simulink model "open_loop_system_modal_kp_kv_int_robustness"  (R2018b)
settings: Solver=ode45  StartTime=0.0  StopTime=10  RelTol=1e-3  EnableMultiTasking=on
values from neighbouring files (symbols this model uses):
  Jpl = 0.0124    [lead_compensator.m]    (also in open_loop_complete_system_analysis.m; poles_placement_kp_kv.m; poles_placement_kp_kv_int.m)
  k = 1    [lead_compensator.m]    (also in poles_placement_kp_kv.m = place(openloop_modal_ss.a,openloop_modal_ss.b,lambda); poles_placement_kp_kv_int.m = place(openloop_modal_int_ss.a,openloop_modal_int_ss.b,lambda)
  km = 0.0235    [lead_compensator.m]    (also in open_loop_complete_system_analysis.m; poles_placement_kp_kv.m; poles_placement_kp_kv_int.m)
settings Model: Creator=c.ponzoni  LastModifiedBy=c.ponzoni
settings DataIOCC: LimitDataPoints=on  SaveFormat=Array
settings OptimizationCC: ExpressionDepthLimit=2147483647  LifeSpan=inf
settings DebuggingCC: UnderspecifiedInitializationDetection=Classic  MergeDetectMultiDrivingBlocksExec=none  StateNameClashWarn=warning  SFUnexpectedBacktrackingDiag=warning  SFNoUnconditionalDefaultTransitionDiag=warning  SFExecutionAtInitializationDiag=none
settings HardwareCC: ProdBitPerPointer=32  ProdBitPerSizeT=32  ProdBitPerPtrDiffT=32  ProdLargestAtomicFloat=None  ProdIntDivRoundTo=Undefined  ProdEndianess=Unspecified  ProdWordSize=32  ProdHWDeviceType=32-bit Generic
settings ModelReferenceCC: PropagateSignalLabelsOutOfModel=off
settings SFSimCC: SimUseLocalCustomCode=off
settings RTWCC: RTWUseLocalCustomCode=off
settings CodeAppCC: StateflowObjectComments=on
settings GRTTargetCC: TargetLangStandard=C89/C90 (ANSI)  GeneratePreprocessorConditionals=Disable all
settings ConfigComp: CovMetricSettings=dw  CovHtmlReporting=on  CovSaveCumulativeToWorkspaceVar=on  CovSaveSingleToWorkspaceVar=on  CovExternalEMLEnable=off

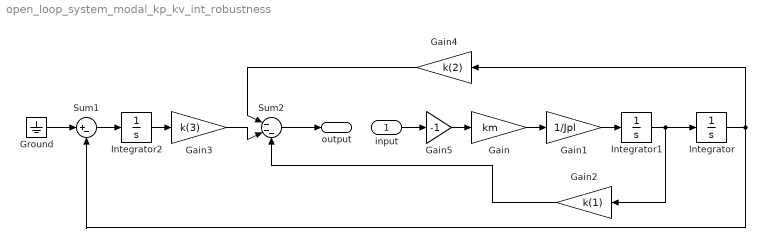
== system open_loop_system_modal_kp_kv_int_robustness ==
  input : Inport
  Gain : Gain  Gain=km  SaturateOnIntegerOverflow=on  OutDataTypeStr=Inherit: Same as input  ParamDataTypeStr=Inherit: Same as input
  Gain1 : Gain  Gain=1/Jpl  SaturateOnIntegerOverflow=on  OutDataTypeStr=Inherit: Same as input  ParamDataTypeStr=Inherit: Same as input
  Gain2 : Gain  Gain=k(1)  SaturateOnIntegerOverflow=on  OutDataTypeStr=Inherit: Same as input  ParamDataTypeStr=Inherit: Same as input
  Gain3 : Gain  Gain=k(3)  SaturateOnIntegerOverflow=on  OutDataTypeStr=Inherit: Same as input  ParamDataTypeStr=Inherit: Same as input
  Gain4 : Gain  Gain=k(2)  SaturateOnIntegerOverflow=on  OutDataTypeStr=Inherit: Same as input  ParamDataTypeStr=Inherit: Same as input
  Gain5 : Gain  Gain=-1  SaturateOnIntegerOverflow=on  OutDataTypeStr=Inherit: Same as input  ParamDataTypeStr=Inherit: Same as input
  Ground : Ground
  Integrator : Integrator
  Integrator1 : Integrator
  Integrator2 : Integrator
  Sum1 : Sum  Inputs=|+-
  Sum2 : Sum  Inputs=|---
  output : Outport
  wires:
  Integrator1/1 -> Gain2/1, Integrator/1
  Gain1/1 -> Integrator1/1
  Gain/1 -> Gain1/1
  Sum1/1 -> Integrator2/1
  Ground/1 -> Sum1/1
  Integrator/1 -> Sum1/2, Gain4/1
  Sum2/1 -> output/1
  Gain2/1 -> Sum2/3
  Gain4/1 -> Sum2/1
  Integrator2/1 -> Gain3/1
  Gain3/1 -> Sum2/2
  input/1 -> Gain5/1
  Gain5/1 -> Gain/1
